simulink model "cukass1"  (R2024a)
settings: Solver=ode4  StartTime=0.0  StopTime=0.3  FixedStep=1e-8  RelTol=1e-3
libraries: spsCurrentMeasurementLib x5, spsSeriesRLCBranchLib x5, spsVoltageMeasurementLib x5, spsDCVoltageSourceLib x1, spsDiodeLib x1, spsMosfetLib x1, simulink x1, sps_lib x1
settings Model: Creator=kotta  LastModifiedBy=User
settings RTWCC: GPUComputeCapability=3.5

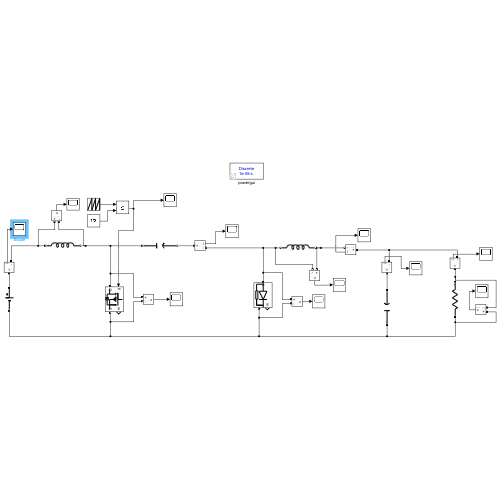
[thumbnail: Simulink's stored preview of the top-level diagram]
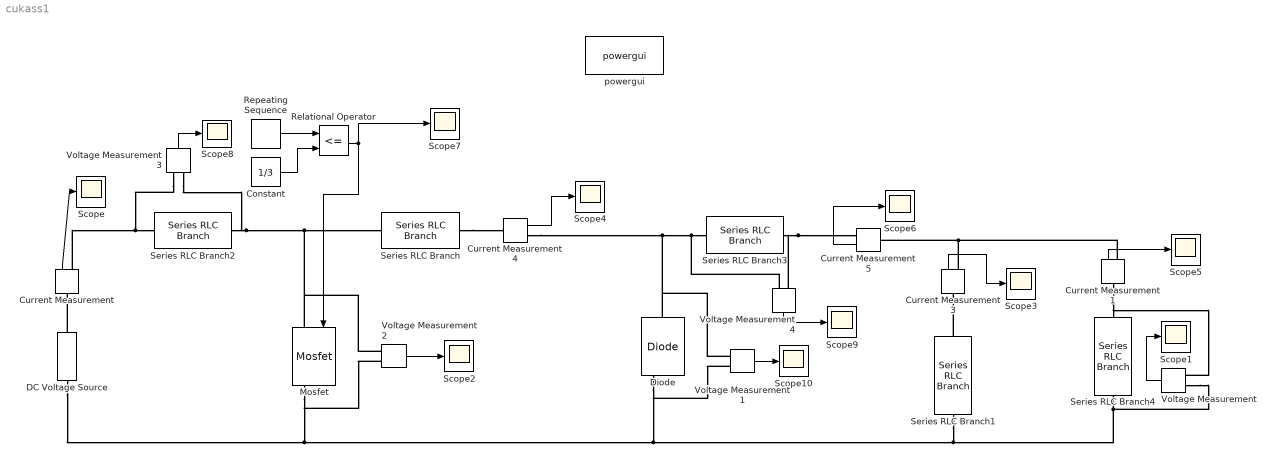
== system cukass1 ==
  Constant : Constant  Value=1/3
  Current Measurement{,1,3..5} (5 alike) : spsCurrentMeasurementLib/Current Measurement  PhasorSimulation=off  OutputType=Complex  PSBequivalent=0
  DC Voltage Source : spsDCVoltageSourceLib/DC Voltage Source  Amplitude=24  Measurements=None
  Diode : spsDiodeLib/Diode  Ron=0.001  Lon=0  Vf=0.8  IC=0  UseSnubber=0  Rs=500  Cs=250e-9  Measurements=on
  Mosfet : spsMosfetLib/Mosfet  Ron=0.01  Lon=0  Rd=0.01  Vfd=0  IC=0  Rs=1e5  Cs=inf  Measurements=on
  Relational Operator : RelationalOperator  Operator=<=  OutDataTypeStr=boolean  RndMeth=Simplest  InputSameDT=off
  Repeating Sequence : simulink/Sources/Repeating Sequence  rep_seq_t=[0 1/100e3]  rep_seq_y=[0 1]
  Scope{,1..10} (11 alike) : Scope
  Series RLC Branch : spsSeriesRLCBranchLib/Series RLC Branch  LConnTagsString=__new0  RConnTagsString=__new0  BranchType=C  Resistance=1  Inductance=1e-3  SetiL0=off  InitialCurrent=0  Capacitance=0.111e-3  Setx0=off  InitialVoltage=36  Measurements=None
  Series RLC Branch1 : spsSeriesRLCBranchLib/Series RLC Branch  LConnTagsString=__new0  RConnTagsString=__new0  BranchType=C  Resistance=1  Inductance=1e-3  SetiL0=off  InitialCurrent=0  Capacitance=25e-6  Setx0=off  InitialVoltage=0  Measurements=None
  Series RLC Branch2 : spsSeriesRLCBranchLib/Series RLC Branch  LConnTagsString=__new0  RConnTagsString=__new0  BranchType=L  Resistance=1  Inductance=0.667e-3  SetiL0=off  InitialCurrent=0  Capacitance=1e-6  Setx0=off  InitialVoltage=0  Measurements=None
  Series RLC Branch3 : spsSeriesRLCBranchLib/Series RLC Branch  LConnTagsString=__new0  RConnTagsString=__new0  BranchType=L  Resistance=1  Inductance=0.333e-3  SetiL0=off  InitialCurrent=0  Capacitance=1e-6  Setx0=off  InitialVoltage=0  Measurements=None
  Series RLC Branch4 : spsSeriesRLCBranchLib/Series RLC Branch  LConnTagsString=__new0  RConnTagsString=__new0  BranchType=R  Resistance=5  Inductance=1e-3  SetiL0=off  InitialCurrent=0  Capacitance=1e-6  Setx0=off  InitialVoltage=0  Measurements=None
  Voltage Measurement{,1..4} (5 alike) : spsVoltageMeasurementLib/Voltage Measurement  PhasorSimulation=off  OutputType=Complex  PSBequivalent=0
  powergui : sps_lib/powergui  Priority=1  SimulationMode=Discrete  SampleTime=1e-8  frequency=60  Iterations=50  frequencyindice=0  Pbase=100e6  ErrMax=1e-4  UnitsV=kV  UnitsW=MW  buscounter=0  FunctionMessages=off  echomessages=off  EnableUseOfTLC=off  CurrentSourceSwitches=off  DisableSnubberDevices=off  DisableRonSwitches=off  DisableVfSwitches=off  DisplayEquations=off  AutomaticDiscreteSolvers=off  SolverType=Tustin/Backward Euler (TBE)  Interpol=off  ExternalGateDelay=off  methode=off  Ts=100  x0status=blocks  SPID=on  SwTol=0  HookPort=off  NonlinearTolerance=1e-4  nMaxIteration=100  ContinueOnMaxIteration=off  RestoreLinks=warning  ResistiveCurrentMeasurement=off  Frange=[0:2:500]  Ylog=off  Xlog=on  ShowGrid=off  save=off  variable=ZData  structure=0  ZoomFFT=off  StartTime=0.0  cycles=1  DisplayStyle=1  fundamental=60  FreqAxis=off  MaxFrequency=1000  frequencyindicesteady=1  RmsSteady=1  display=off
  wires:
  Repeating Sequence/1 -> Relational Operator/1
  Constant/1 -> Relational Operator/2
  Relational Operator/1 -> Mosfet/1, Scope7/1
  Current Measurement4/1 -> Scope4/1
  Voltage Measurement2/1 -> Scope2/1
  Current Measurement/1 -> Scope/1
  Current Measurement3/1 -> Scope3/1
  Current Measurement5/1 -> Scope6/1
  Voltage Measurement/1 -> Scope1/1
  Current Measurement1/1 -> Scope5/1
  Voltage Measurement4/1 -> Scope9/1
  Voltage Measurement3/1 -> Scope8/1
  Voltage Measurement1/1 -> Scope10/1
  connections:
  DC Voltage Source/RConn1 -- Current Measurement/LConn1
  Current Measurement/RConn1 -- Voltage Measurement3/LConn1 -- Series RLC Branch2/LConn1
  Series RLC Branch2/RConn1 -- Voltage Measurement2/LConn1 -- Mosfet/LConn1 -- Series RLC Branch/LConn1 -- Voltage Measurement3/LConn2
  Series RLC Branch/RConn1 -- Current Measurement4/LConn1
  Current Measurement4/RConn1 -- Voltage Measurement1/LConn1 -- Diode/LConn1 -- Voltage Measurement4/LConn2 -- Series RLC Branch3/LConn1
  Current Measurement3/RConn1 -- Current Measurement5/LConn1 -- Current Measurement1/RConn1
  Series RLC Branch4/LConn1 -- Voltage Measurement/LConn2 -- Current Measurement1/LConn1
  DC Voltage Source/LConn1 -- Voltage Measurement2/LConn2 -- Mosfet/RConn1 -- Voltage Measurement1/LConn2 -- Diode/RConn1 -- Voltage Measurement/LConn1 -- Series RLC Branch4/RConn1 -- Series RLC Branch1/LConn1
  Series RLC Branch3/RConn1 -- Current Measurement5/RConn1 -- Voltage Measurement4/LConn1
  Series RLC Branch1/RConn1 -- Current Measurement3/LConn1
